simulink model "Hw6P1a"  (R2017a)
settings: Solver=FixedStepAuto  StartTime=0.0  StopTime=10.0  FixedStep=0.01  RelTol=1e-3
values from neighbouring files (symbols this model uses):
  w = 0    [Hw6P1.m]
libraries: fuzblock x4
settings Model: Creator=Soutrik  LastModifiedBy=Soutrik

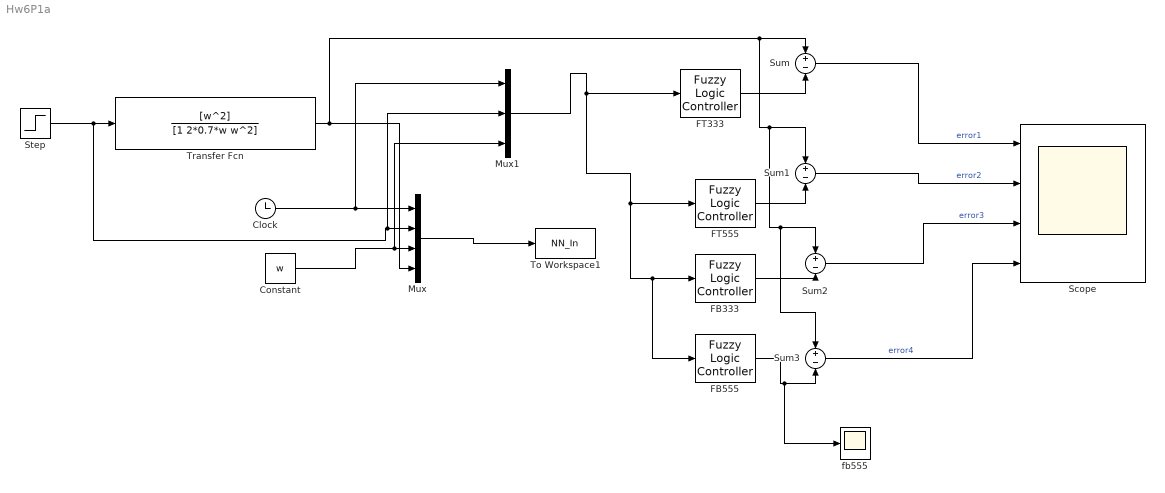
== system Hw6P1a ==
  Clock : Clock
  Constant : Constant  Value=w
  FB333 : fuzblock/Fuzzy Logic  Controller  fis=fb333
  FB555 : fuzblock/Fuzzy Logic  Controller  fis=fb555
  FT333 : fuzblock/Fuzzy Logic  Controller  fis=ft333
  FT555 : fuzblock/Fuzzy Logic  Controller  fis=ft555
  Mux : Mux
  Mux1 : Mux  Inputs=3
  Scope : Scope  NumInputPorts=4
  Step : Step  SampleTime=0
  Sum{,1..3} (4 alike) : Sum  Inputs=+-
  To Workspace1 : ToWorkspace  VariableName=NN_In  SampleTime=-1
  Transfer Fcn : TransferFcn  Numerator=[w^2]  Denominator=[1 2*0.7*w w^2]
  fb555 : Scope
  wires:
  Step/1 -> Mux1/2, Mux/2, Transfer Fcn/1
  Clock/1 -> Mux1/1, Mux/1
  Constant/1 -> Mux1/3, Mux/3
  Mux/1 -> To Workspace1/1
  Transfer Fcn/1 -> Sum3/1, Sum2/1, Sum1/1, Sum/1, Mux/4
  Mux1/1 -> FB555/1, FB333/1, FT555/1, FT333/1
  FT333/1 -> Sum/2
  FT555/1 -> Sum1/2
  FB333/1 -> Sum2/2
  FB555/1 -> fb555/1, Sum3/2
  Sum/1 -> Scope/1  "error1"
  Sum1/1 -> Scope/2  "error2"
  Sum2/1 -> Scope/3  "error3"
  Sum3/1 -> Scope/4  "error4"
